simulink model "simu"  (R2021a)
settings: Solver=VariableStepAuto  StartTime=0.0  StopTime=15  MaxStep=0.1  RelTol=1e-3
values from neighbouring files (symbols this model uses):
  a = 0.86    [ProjetoControleTanqueConicoFinal.m]    (also in TrabalhoTanqueConico.m = 4*A2*sqrt(2*g)/(pi*0.6^2); TrabalhoTanqueConicoOutraVersao.m = 4*A2*sqrt(2*g)/(pi*0.6^2))
  b = 3.53    [ProjetoControleTanqueConicoFinal.m]    (also in TrabalhoTanqueConico.m = 3.53677651315; TrabalhoTanqueConicoOutraVersao.m = 3.53677651315)
  d = 0.6    [ProjetoControleTanqueConicoFinal.m]
  hbar = 6    [ProjetoControleTanqueConicoFinal.m]    (also in TrabalhoTanqueConico.m = 5; TrabalhoTanqueConicoOutraVersao.m = 5)
  k1 = K(1,1)    [ProjetoControleTanqueConicoFinal.m]
  k2 = K(1,2)    [ProjetoControleTanqueConicoFinal.m]
settings Model: Creator=danie  LastModifiedBy=guilh
settings SolverCC: AlgebraicLoopSolver=TrustRegion
settings DataIOCC: ReturnWorkspaceOutputs=off
settings DebuggingCC: SFMachineParentedDataDiag=warning  ArithmeticOperatorsInVariantConditions=warning
settings SFSimCC: SimUseLocalCustomCode=off  CustomCodeUndefinedFunction=UseInterfaceOnly
settings RTWCC: RTWUseLocalCustomCode=off

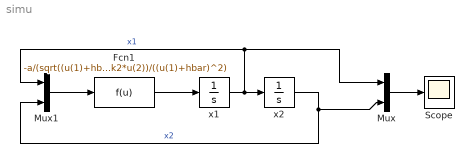
== system simu ==
  Fcn1 : Fcn  Expr=-a/(sqrt((u(1)+hbar)^3)) + b*d/((u(1)+hbar)^2)+b*(k1*u(1)+k2*u(2))/((u(1)+hbar)^2)
  Mux : Mux  Inputs=2
  Mux1 : Mux  Inputs=2
  Scope : Scope
  x1 : Integrator  InitialCondition=1
  x2 : Integrator  InitialCondition=1
  wires:
  x1/1 -> Mux1/1, Mux/1, x2/1  "x1"
  Fcn1/1 -> x1/1
  Mux1/1 -> Fcn1/1
  x2/1 -> Mux/2, Mux1/2  "x2"
  Mux/1 -> Scope/1
